simulink library "Loudness"  (R2022b)
settings: Solver=VariableStepAuto  StartTime=0.0  StopTime=10.0  RelTol=1e-3
InitFcn:
  | Loudness_init;
values from neighbouring files (symbols this model uses):
  COMP = struct('zipCoef', COMP_zipCoef,      'LoudBPFNum', COMPBASS_Num, 'LoudBPFDenom', COMPBASS_Denom,      'LoudLPFNum', COMPMID_Num, 'LoudLPFDenom', COMPMID_Denom,      'LoudBPFFreq',COMPBASS_Fc,'LoudBPFQ',COMPBASS_Q,      'LoudLPFFreq',COMPMID_Fc,'LoudLPFQ',COMPMID_Q)    [Loudness_init.m]
undefined symbols (not defined in the file or in its folder): dfilt, LOUD_BASS_0DB_SCALE, LOUD_BASS_D1, LOUD_BASS_D2, sys_defs
libraries: TuneVar x38, RTC x16, dspobslib x5
(part 2 of 2)

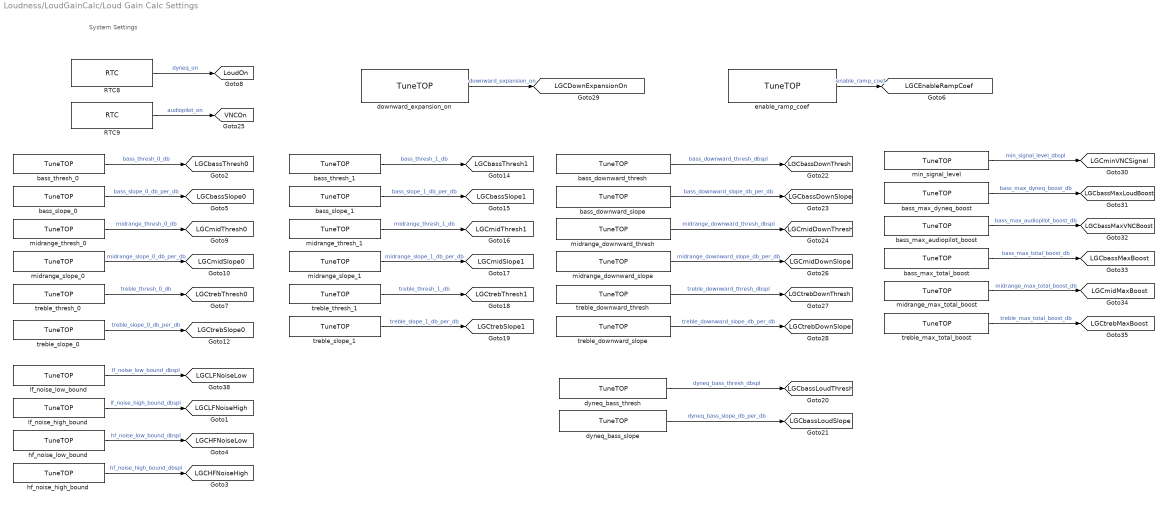
== system Loudness/LoudGainCalc/Loud Gain Calc Settings ==
  note: System Settings
  RTC8 : RTC/RTC  REQ_Priority=RTC_Mask.NormalPriority  RequestAtInit=off  EnableRequest=off  REQElemName1=dyneq_on  REQElemType1=single  REQElemWidth1=1  REQElemInitial1=[]  REQElemType2=single  REQElemWidth2=1  REQElemInitial2=[]  REQElemType3=uint32  REQElemWidth3=1  REQElemInitial3=[]  REQElemType4=uint32  REQElemWidth4=1  REQElemInitial4=[]  REQElemType5=uint32  REQElemWidth5=1  REQElemInitial5=[]  REQElemType6=uint32  REQElemWidth6=1  REQElemInitial6=[]  REQElemType7=uint32  REQElemWidth7=1  REQElemInitial7=[]  REQElemType8=uint32  REQElemWidth8=1  REQElemInitial8=[]  REQElemType9=uint32  REQElemWidth9=1  REQElemInitial9=[]  REQElemType10=uint32  REQElemWidth10=1  REQElemInitial10=[]  EnableResponse=off  EnableRSP_StatusIn=off  RSPElemType1=uint32  RSPElemWidth1=1  RSPElemType2=uint32  RSPElemWidth2=1  RSPElemType3=uint32  RSPElemWidth3=1  RSPElemType4=uint32  RSPElemWidth4=1  RSPElemType5=uint32  RSPElemWidth5=1  RSPElemType6=uint32  RSPElemWidth6=1  RSPElemType7=uint32  RSPElemWidth7=1  RSPElemType8=uint32  RSPElemWidth8=1  RSPElemType9=uint32  RSPElemWidth9=1  RSPElemType10=uint32  RSPElemWidth10=1  EnableNotification=off  EnableNTF_PrepTrig=off  NTFElemType1=uint32  NTFElemWidth1=1  NTFElemType2=uint32  NTFElemWidth2=1  NTFElemType3=uint32  NTFElemWidth3=1  NTFElemType4=uint32  NTFElemWidth4=1  NTFElemType5=uint32  NTFElemWidth5=1  NTFElemType6=uint32  NTFElemWidth6=1  NTFElemType7=uint32  NTFElemWidth7=1  NTFElemType8=uint32  NTFElemWidth8=1  NTFElemType9=uint32  NTFElemWidth9=1  NTFElemType10=uint32  NTFElemWidth10=1  MaskMessageName=setDyneqOn
  RTC9 : RTC/RTC  REQ_Priority=RTC_Mask.NormalPriority  RequestAtInit=off  EnableRequest=off  REQElemName1=audiopilot_on  REQElemType1=single  REQElemWidth1=1  REQElemInitial1=[]  REQElemType2=single  REQElemWidth2=1  REQElemInitial2=[]  REQElemType3=uint32  REQElemWidth3=1  REQElemInitial3=[]  REQElemType4=uint32  REQElemWidth4=1  REQElemInitial4=[]  REQElemType5=uint32  REQElemWidth5=1  REQElemInitial5=[]  REQElemType6=uint32  REQElemWidth6=1  REQElemInitial6=[]  REQElemType7=uint32  REQElemWidth7=1  REQElemInitial7=[]  REQElemType8=uint32  REQElemWidth8=1  REQElemInitial8=[]  REQElemType9=uint32  REQElemWidth9=1  REQElemInitial9=[]  REQElemType10=uint32  REQElemWidth10=1  REQElemInitial10=[]  EnableResponse=off  EnableRSP_StatusIn=off  RSPElemType1=uint32  RSPElemWidth1=1  RSPElemType2=uint32  RSPElemWidth2=1  RSPElemType3=uint32  RSPElemWidth3=1  RSPElemType4=uint32  RSPElemWidth4=1  RSPElemType5=uint32  RSPElemWidth5=1  RSPElemType6=uint32  RSPElemWidth6=1  RSPElemType7=uint32  RSPElemWidth7=1  RSPElemType8=uint32  RSPElemWidth8=1  RSPElemType9=uint32  RSPElemWidth9=1  RSPElemType10=uint32  RSPElemWidth10=1  EnableNotification=off  EnableNTF_PrepTrig=off  NTFElemType1=uint32  NTFElemWidth1=1  NTFElemType2=uint32  NTFElemWidth2=1  NTFElemType3=uint32  NTFElemWidth3=1  NTFElemType4=uint32  NTFElemWidth4=1  NTFElemType5=uint32  NTFElemWidth5=1  NTFElemType6=uint32  NTFElemWidth6=1  NTFElemType7=uint32  NTFElemWidth7=1  NTFElemType8=uint32  NTFElemWidth8=1  NTFElemType9=uint32  NTFElemWidth9=1  NTFElemType10=uint32  NTFElemWidth10=1  MaskMessageName=setAudioPilotOn
  bass_downward_slope : TuneVar/TuneTOP  TriggerInit=[-60 184 115 216]  TopName=bass_downward_slope_db_per_db  TuneName=bass_downward_slope_db_per_db  DataType=Inherit: Same as input  PackageName=mode  BankNumber=0  TunabilityNumber=1  MinValue=[]  MaxValue=[]  UseSameName=on  MaskValue=single([LGC.bassDownSlope])
  bass_downward_thresh : TuneVar/TuneTOP  TriggerInit=[-60 135 115 165]  TopName=bass_downward_thresh_dbspl  TuneName=bass_downward_thresh_dbspl  DataType=Inherit: Same as input  PackageName=mode  BankNumber=0  TunabilityNumber=1  MinValue=[]  MaxValue=[]  UseSameName=on  MaskValue=single([LGC.bassDownThresh])
  bass_max_audiopilot_boost : TuneVar/TuneTOP  TriggerInit=[445 230 605 260]  TopName=bass_max_audiopilot_boost_db  TuneName=bass_max_audiopilot_boost_db  DataType=Inherit: Same as input  PackageName=mode  BankNumber=0  TunabilityNumber=1  MinValue=[]  MaxValue=[]  UseSameName=on  MaskValue=single([LGC.bassMaxVNCBoost])
  bass_max_dyneq_boost : TuneVar/TuneTOP  TriggerInit=[445 179 605 211]  TopName=bass_max_dyneq_boost_db  TuneName=bass_max_dyneq_boost_db  DataType=Inherit: Same as input  PackageName=mode  BankNumber=0  TunabilityNumber=1  MinValue=[]  MaxValue=[]  UseSameName=on  MaskValue=single([LGC.bassMaxLoudBoost])
  bass_max_total_boost : TuneVar/TuneTOP  TriggerInit=[445 279 605 311]  TopName=bass_max_total_boost_db  TuneName=bass_max_total_boost_db  DataType=Inherit: Same as input  PackageName=mode  BankNumber=0  TunabilityNumber=1  MinValue=[]  MaxValue=[]  UseSameName=on  MaskValue=single([LGC.bassMaxBoost])
  bass_slope_0 : TuneVar/TuneTOP  TriggerInit=[-895 185 -755 215]  TopName=bass_slope_0_db_per_db  TuneName=bass_slope_0_db_per_db  DataType=Inherit: Same as input  PackageName=mode  BankNumber=0  TunabilityNumber=1  MinValue=[]  MaxValue=[]  UseSameName=on  MaskValue=single([LGC.bassSlope0])
  bass_slope_1 : TuneVar/TuneTOP  TriggerInit=[-470 185 -330 215]  TopName=bass_slope_1_db_per_db  TuneName=bass_slope_1_db_per_db  DataType=Inherit: Same as input  PackageName=mode  BankNumber=0  TunabilityNumber=1  MinValue=[]  MaxValue=[]  UseSameName=on  MaskValue=single([LGC.bassSlope1])
  bass_thresh_0 : TuneVar/TuneTOP  TriggerInit=[-895 135 -755 165]  TopName=bass_thresh_0_db  TuneName=bass_thresh_0_db  DataType=Inherit: Same as input  PackageName=mode  BankNumber=0  TunabilityNumber=1  MinValue=[]  MaxValue=[]  UseSameName=on  MaskValue=single([LGC.bassThresh0])
  bass_thresh_1 : TuneVar/TuneTOP  TriggerInit=[-470 135 -330 165]  TopName=bass_thresh_1_db  TuneName=bass_thresh_1_db  DataType=Inherit: Same as input  PackageName=mode  BankNumber=0  TunabilityNumber=1  MinValue=[]  MaxValue=[]  UseSameName=on  MaskValue=single([LGC.bassThresh1])
  downward_expansion_on : TuneVar/TuneTOP  TriggerInit=[-360 5 -195 55]  TopName=downward_expansion_on  TuneName=downward_expansion_on  DataType=Inherit: Same as input  PackageName=mode  BankNumber=0  TunabilityNumber=1  MinValue=[]  MaxValue=[]  UseSameName=on  MaskValue=single([LGC.downward_expansion_on])
  dyneq_bass_slope : TuneVar/TuneTOP  TriggerInit=[-55 529 110 561]  TopName=dyneq_bass_slope_db_per_db  TuneName=dyneq_bass_slope_db_per_db  DataType=Inherit: Same as input  PackageName=mode  BankNumber=0  TunabilityNumber=1  MinValue=[]  MaxValue=[]  UseSameName=on  MaskValue=single([LGC.bassLoudSlope])
  dyneq_bass_thresh : TuneVar/TuneTOP  TriggerInit=[-55 479 110 511]  TopName=dyneq_bass_thresh_dbspl  TuneName=dyneq_bass_thresh_dbspl  DataType=Inherit: Same as input  PackageName=mode  BankNumber=0  TunabilityNumber=1  MinValue=[]  MaxValue=[]  UseSameName=on  MaskValue=single([LGC.bassLoudThresh])
  enable_ramp_coef : TuneVar/TuneTOP  TriggerInit=[205 5 370 55]  TopName=enable_ramp_coef  TuneName=enable_ramp_coef  DataType=Inherit: Same as input  PackageName=mode  BankNumber=0  TunabilityNumber=1  MinValue=[]  MaxValue=[]  UseSameName=on  MaskValue=single(LGC.enableRampCoef)
  hf_noise_high_bound : TuneVar/TuneTOP  TriggerInit=[-895 610 -755 640]  TopName=hf_noise_high_bound_dbspl  TuneName=hf_noise_high_bound_dbspl  DataType=Inherit: Same as input  PackageName=mode  BankNumber=0  TunabilityNumber=1  MinValue=[]  MaxValue=[]  UseSameName=on  MaskValue=single([LGC.HFNoiseHigh])
  hf_noise_low_bound : TuneVar/TuneTOP  TriggerInit=[-895 560 -755 590]  TopName=hf_noise_low_bound_dbspl  TuneName=hf_noise_low_bound_dbspl  DataType=Inherit: Same as input  PackageName=mode  BankNumber=0  TunabilityNumber=1  MinValue=[]  MaxValue=[]  UseSameName=on  MaskValue=single([LGC.HFNoiseLow])
  lf_noise_high_bound : TuneVar/TuneTOP  TriggerInit=[-895 510 -755 540]  TopName=lf_noise_high_bound_dbspl  TuneName=lf_noise_high_bound_dbspl  DataType=Inherit: Same as input  PackageName=mode  BankNumber=0  TunabilityNumber=1  MinValue=[]  MaxValue=[]  UseSameName=on  MaskValue=single([LGC.LFNoiseHigh])
  lf_noise_low_bound : TuneVar/TuneTOP  TriggerInit=[-895 460 -755 490]  TopName=lf_noise_low_bound_dbspl  TuneName=lf_noise_low_bound_dbspl  DataType=Inherit: Same as input  PackageName=mode  BankNumber=0  TunabilityNumber=1  MinValue=[]  MaxValue=[]  UseSameName=on  MaskValue=single([LGC.LFNoiseLow])
  midrange_downward_slope : TuneVar/TuneTOP  TriggerInit=[-60 285 115 315]  TopName=midrange_downward_slope_db_per_db  TuneName=midrange_downward_slope_db_per_db  DataType=Inherit: Same as input  PackageName=mode  BankNumber=0  TunabilityNumber=1  MinValue=[]  MaxValue=[]  UseSameName=on  MaskValue=single([LGC.midDownSlope])
  midrange_downward_thresh : TuneVar/TuneTOP  TriggerInit=[-60 234 115 266]  TopName=midrange_downward_thresh_dbspl  TuneName=midrange_downward_thresh_dbspl  DataType=Inherit: Same as input  PackageName=mode  BankNumber=0  TunabilityNumber=1  MinValue=[]  MaxValue=[]  UseSameName=on  MaskValue=single([LGC.midDownThresh])
  midrange_max_total_boost : TuneVar/TuneTOP  TriggerInit=[445 331 605 359]  TopName=midrange_max_total_boost_db  TuneName=midrange_max_total_boost_db  DataType=Inherit: Same as input  PackageName=mode  BankNumber=0  TunabilityNumber=1  MinValue=[]  MaxValue=[]  UseSameName=on  MaskValue=single([LGC.midMaxBoost])
  midrange_slope_0 : TuneVar/TuneTOP  TriggerInit=[-895 285 -755 315]  TopName=midrange_slope_0_db_per_db  TuneName=midrange_slope_0_db_per_db  DataType=Inherit: Same as input  PackageName=mode  BankNumber=0  TunabilityNumber=1  MinValue=[]  MaxValue=[]  UseSameName=on  MaskValue=single([LGC.midSlope0])
  midrange_slope_1 : TuneVar/TuneTOP  TriggerInit=[-470 285 -330 315]  TopName=midrange_slope_1_db_per_db  TuneName=midrange_slope_1_db_per_db  DataType=Inherit: Same as input  PackageName=mode  BankNumber=0  TunabilityNumber=1  MinValue=[]  MaxValue=[]  UseSameName=on  MaskValue=single([LGC.midSlope1])
  midrange_thresh_0 : TuneVar/TuneTOP  TriggerInit=[-895 235 -755 265]  TopName=midrange_thresh_0_db  TuneName=midrange_thresh_0_db  DataType=Inherit: Same as input  PackageName=mode  BankNumber=0  TunabilityNumber=1  MinValue=[]  MaxValue=[]  UseSameName=on  MaskValue=single([LGC.midThresh0])
  midrange_thresh_1 : TuneVar/TuneTOP  TriggerInit=[-470 235 -330 265]  TopName=midrange_thresh_1_db  TuneName=midrange_thresh_1_db  DataType=Inherit: Same as input  PackageName=mode  BankNumber=0  TunabilityNumber=1  MinValue=[]  MaxValue=[]  UseSameName=on  MaskValue=single([LGC.midThresh1])
  min_signal_level : TuneVar/TuneTOP  TriggerInit=[445 131 605 159]  TopName=min_signal_level_dbspl  TuneName=min_signal_level_dbspl  DataType=Inherit: Same as input  PackageName=mode  BankNumber=0  TunabilityNumber=1  MinValue=[]  MaxValue=[]  UseSameName=on  MaskValue=single([LGC.minVNCSignal])
  treble_downward_slope : TuneVar/TuneTOP  TriggerInit=[-60 385 115 415]  TopName=treble_downward_slope_db_per_db  TuneName=treble_downward_slope_db_per_db  DataType=Inherit: Same as input  PackageName=mode  BankNumber=0  TunabilityNumber=1  MinValue=[]  MaxValue=[]  UseSameName=on  MaskValue=single([LGC.trebDownSlope])
  treble_downward_thresh : TuneVar/TuneTOP  TriggerInit=[-60 336 115 364]  TopName=treble_downward_thresh_dbspl  TuneName=treble_downward_thresh_dbspl  DataType=Inherit: Same as input  PackageName=mode  BankNumber=0  TunabilityNumber=1  MinValue=[]  MaxValue=[]  UseSameName=on  MaskValue=single([LGC.trebDownThresh])
  treble_max_total_boost : TuneVar/TuneTOP  TriggerInit=[445 380 605 410]  TopName=treble_max_total_boost_db  TuneName=treble_max_total_boost_db  DataType=Inherit: Same as input  PackageName=mode  BankNumber=0  TunabilityNumber=1  MinValue=[]  MaxValue=[]  UseSameName=on  MaskValue=single([LGC.trebMaxBoost])
  treble_slope_0 : TuneVar/TuneTOP  TriggerInit=[-895 390 -755 420]  TopName=treble_slope_0_db_per_db  TuneName=treble_slope_0_db_per_db  DataType=Inherit: Same as input  PackageName=mode  BankNumber=0  TunabilityNumber=1  MinValue=[]  MaxValue=[]  UseSameName=on  MaskValue=single([LGC.trebSlope0])
  treble_slope_1 : TuneVar/TuneTOP  TriggerInit=[-470 385 -330 415]  TopName=treble_slope_1_db_per_db  TuneName=treble_slope_1_db_per_db  DataType=Inherit: Same as input  PackageName=mode  BankNumber=0  TunabilityNumber=1  MinValue=[]  MaxValue=[]  UseSameName=on  MaskValue=single([LGC.trebSlope1])
  treble_thresh_0 : TuneVar/TuneTOP  TriggerInit=[-895 335 -755 365]  TopName=treble_thresh_0_db  TuneName=treble_thresh_0_db  DataType=Inherit: Same as input  PackageName=mode  BankNumber=0  TunabilityNumber=1  MinValue=[]  MaxValue=[]  UseSameName=on  MaskValue=single([LGC.trebThresh0])
  treble_thresh_1 : TuneVar/TuneTOP  TriggerInit=[-470 335 -330 365]  TopName=treble_thresh_1_db  TuneName=treble_thresh_1_db  DataType=Inherit: Same as input  PackageName=mode  BankNumber=0  TunabilityNumber=1  MinValue=[]  MaxValue=[]  UseSameName=on  MaskValue=single([LGC.trebThresh1])
  tag scope: LGCDownExpansionOn=global, LGCEnableRampCoef=global, LGCHFNoiseHigh=global, LGCHFNoiseLow=global, LGCLFNoiseHigh=global, LGCLFNoiseLow=global, LGCbassDownSlope=global, LGCbassDownThresh=global, LGCbassLoudSlope=global, LGCbassLoudThresh=global, LGCbassMaxBoost=global, LGCbassMaxLoudBoost=global, LGCbassMaxVNCBoost=global, LGCbassSlope0=global, LGCbassSlope1=global, LGCbassThresh0=global, LGCbassThresh1=global, LGCmidDownSlope=global, LGCmidDownThresh=global, LGCmidMaxBoost=global, LGCmidSlope0=global, LGCmidSlope1=global, LGCmidThresh0=global, LGCmidThresh1=global, LGCminVNCSignal=global, LGCtrebDownSlope=global, LGCtrebDownThresh=global, LGCtrebMaxBoost=global, LGCtrebSlope0=global, LGCtrebSlope1=global, LGCtrebThresh0=global, LGCtrebThresh1=global, LoudOn=global, VNCOn=global
  wires:
  lf_noise_low_bound/1 -> [LGCLFNoiseLow]  "lf_noise_low_bound_dbspl"
  lf_noise_high_bound/1 -> [LGCLFNoiseHigh]  "lf_noise_high_bound_dbspl"
  bass_thresh_0/1 -> [LGCbassThresh0]  "bass_thresh_0_db"
  bass_slope_0/1 -> [LGCbassSlope0]  "bass_slope_0_db_per_db"
  treble_thresh_0/1 -> [LGCtrebThresh0]  "treble_thresh_0_db"
  midrange_thresh_0/1 -> [LGCmidThresh0]  "midrange_thresh_0_db"
  midrange_slope_0/1 -> [LGCmidSlope0]  "midrange_slope_0_db_per_db"
  treble_slope_0/1 -> [LGCtrebSlope0]  "treble_slope_0_db_per_db"
  bass_thresh_1/1 -> [LGCbassThresh1]  "bass_thresh_1_db"
  bass_slope_1/1 -> [LGCbassSlope1]  "bass_slope_1_db_per_db"
  midrange_thresh_1/1 -> [LGCmidThresh1]  "midrange_thresh_1_db"
  midrange_slope_1/1 -> [LGCmidSlope1]  "midrange_slope_1_db_per_db"
  treble_slope_1/1 -> [LGCtrebSlope1]  "treble_slope_1_db_per_db"
  dyneq_bass_thresh/1 -> [LGCbassLoudThresh]  "dyneq_bass_thresh_dbspl"
  dyneq_bass_slope/1 -> [LGCbassLoudSlope]  "dyneq_bass_slope_db_per_db"
  bass_downward_thresh/1 -> [LGCbassDownThresh]  "bass_downward_thresh_dbspl"
  bass_downward_slope/1 -> [LGCbassDownSlope]  "bass_downward_slope_db_per_db"
  midrange_downward_thresh/1 -> [LGCmidDownThresh]  "midrange_downward_thresh_dbspl"
  midrange_downward_slope/1 -> [LGCmidDownSlope]  "midrange_downward_slope_db_per_db"
  treble_downward_thresh/1 -> [LGCtrebDownThresh]  "treble_downward_thresh_dbspl"
  treble_downward_slope/1 -> [LGCtrebDownSlope]  "treble_downward_slope_db_per_db"
  min_signal_level/1 -> [LGCminVNCSignal]  "min_signal_level_dbspl"
  bass_max_dyneq_boost/1 -> [LGCbassMaxLoudBoost]  "bass_max_dyneq_boost_db"
  bass_max_audiopilot_boost/1 -> [LGCbassMaxVNCBoost]  "bass_max_audiopilot_boost_db"
  bass_max_total_boost/1 -> [LGCbassMaxBoost]  "bass_max_total_boost_db"
  midrange_max_total_boost/1 -> [LGCmidMaxBoost]  "midrange_max_total_boost_db"
  treble_max_total_boost/1 -> [LGCtrebMaxBoost]  "treble_max_total_boost_db"
  downward_expansion_on/1 -> [LGCDownExpansionOn]  "downward_expansion_on"
  treble_thresh_1/1 -> [LGCtrebThresh1]  "treble_thresh_1_db"
  hf_noise_low_bound/1 -> [LGCHFNoiseLow]  "hf_noise_low_bound_dbspl"
  hf_noise_high_bound/1 -> [LGCHFNoiseHigh]  "hf_noise_high_bound_dbspl"
  RTC8/1 -> [LoudOn]  "dyneq_on"
  RTC9/1 -> [VNCOn]  "audiopilot_on"
  enable_ramp_coef/1 -> [LGCEnableRampCoef]  "enable_ramp_coef"

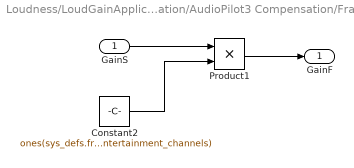
== system Loudness/LoudGainApplication/AudioPilot3 Compensation/Framify ==
  GainS : Inport
  Constant2 : Constant  Value=ones(sys_defs.frameSize, sys_defs.number_of_input_entertainment_channels)  VectorParams1D=off  OutDataTypeStr=single
  Product1 : Product  RndMeth=Zero
  GainF : Outport  VectorParamsAs1DForOutWhenUnconnected=off
  wires:
  Product1/1 -> GainF/1
  Constant2/1 -> Product1/2
  GainS/1 -> Product1/1

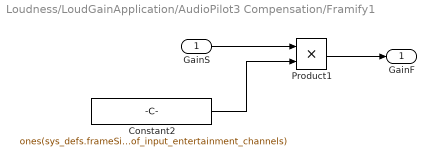
== system Loudness/LoudGainApplication/AudioPilot3 Compensation/Framify1 ==
  GainS : Inport  OutDataTypeStr=single
  Constant2 : Constant  Value=ones(sys_defs.frameSize, sys_defs.number_of_input_entertainment_channels)  VectorParams1D=off  OutDataTypeStr=single
  Product1 : Product  RndMeth=Zero
  GainF : Outport  VectorParamsAs1DForOutWhenUnconnected=off
  wires:
  GainS/1 -> Product1/1
  Constant2/1 -> Product1/2
  Product1/1 -> GainF/1

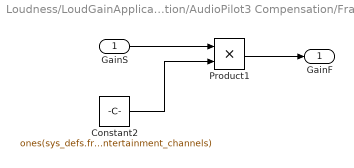
== system Loudness/LoudGainApplication/AudioPilot3 Compensation/Framify2 ==
  GainS : Inport
  Constant2 : Constant  Value=ones(sys_defs.frameSize, sys_defs.number_of_input_entertainment_channels)  VectorParams1D=off  OutDataTypeStr=single
  Product1 : Product  RndMeth=Zero
  GainF : Outport  VectorParamsAs1DForOutWhenUnconnected=off
  wires:
  Product1/1 -> GainF/1
  Constant2/1 -> Product1/2
  GainS/1 -> Product1/1

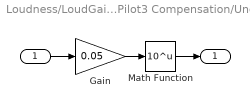
== system Loudness/LoudGainApplication/AudioPilot3 Compensation/UndB ==
  " " : Inport
  Gain : Gain  Gain=0.05  SaturateOnIntegerOverflow=on  OutDataTypeStr=Inherit: Same as input  ParamDataTypeStr=Inherit: Same as input
  Math Function : Math  Operator=10^u  SignedPower=on
  "  " : Outport  VectorParamsAs1DForOutWhenUnconnected=off
  wires:
  Gain/1 -> Math Function/1
  Math Function/1 -> "  "/1
  " "/1 -> Gain/1

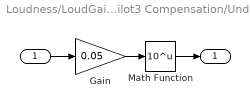
== system Loudness/LoudGainApplication/AudioPilot3 Compensation/UndB1 ==
  " " : Inport
  Gain : Gain  Gain=0.05  SaturateOnIntegerOverflow=on  OutDataTypeStr=Inherit: Same as input  ParamDataTypeStr=Inherit: Same as input
  Math Function : Math  Operator=10^u  SignedPower=on
  "  " : Outport  VectorParamsAs1DForOutWhenUnconnected=off
  wires:
  " "/1 -> Gain/1
  Math Function/1 -> "  "/1
  Gain/1 -> Math Function/1

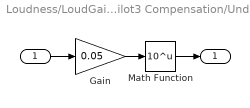
== system Loudness/LoudGainApplication/AudioPilot3 Compensation/UndB2 ==
  " " : Inport
  Gain : Gain  Gain=0.05  SaturateOnIntegerOverflow=on  OutDataTypeStr=Inherit: Same as input  ParamDataTypeStr=Inherit: Same as input
  Math Function : Math  Operator=10^u  SignedPower=on
  "  " : Outport  VectorParamsAs1DForOutWhenUnconnected=off
  wires:
  " "/1 -> Gain/1
  Math Function/1 -> "  "/1
  Gain/1 -> Math Function/1

== matlab function Loudness/LoudGainCalc/Boost Map Adjustments ==
  data: Bthresh output; Bslope output; noise input; LFNoiseLow input; LFNoiseHigh input; HFNoiseLow input; HFNoiseHigh input; ratio input; ratioLow input; ratioHigh input; BT0 input; BS0 input; MT0 input; MS0 input; TT0 input; TS0 input; BT1 input; BS1 input; MT1 input; MS1 input; TT1 input; Mthresh output; Mslope output; TS1 input; Tthresh output; Tslope output; HFNoise input
function [Bthresh, Bslope, Mthresh, Mslope, Tthresh ,Tslope] = ...
	fcn(noise, ...
	LFNoiseLow, LFNoiseHigh, ...
	HFNoiseLow, HFNoiseHigh, ...
    ratio, ratioLow, ratioHigh, ...
	BT0, BS0, MT0, MS0, TT0, TS0, ...
	BT1, BS1, MT1, MS1, TT1, TS1,HFNoise)
% This block supports an embeddable subset of the MATLAB language.
% See the help menu for details. 

% Initializing the parameters
% Concatenate ratioHigh & ratioLow to form ratio0
ratio0 = [ratioHigh ratioLow];
% Concatenate BT0 & BT1 to form Bthresh0
Bthresh0 = [BT0 BT1];
% Concatenate MT0 & MT1 to form Mthresh0
Mthresh0 = [MT0 MT1];
% Concatenate TT0 & TT1 to form Tthresh0
Tthresh0 = [TT0 TT1];
% Concatenate BS0 & BS1 to form Bslope0
Bslope0 = [BS0 BS1];
% Concatenate MS0 & MS1 to form Mslope0
Mslope0 = [MS0 MS1];
% Concatenate TS0 & TS1 to form Tslope0
Tslope0 = [TS0 TS1];
% Assign Value for alpha based on HFNoise, HFNoiseLow & HFNoiseHigh values
if HFNoise < HFNoiseLow
    alpha = single(0);
elseif HFNoise > HFNoiseHigh
    alpha = single(1);
else
    alpha = single((HFNoise-HFNoiseLow)/(HFNoiseHigh-HFNoiseLow));
end
% Assign Value for beta based on noise, LFNoiseLow & LFNoiseHigh values
if noise < LFNoiseLow
    beta = single(0);
elseif noise > LFNoiseHigh
    beta = single(1);
else
    beta  = single((noise-LFNoiseLow)/(LFNoiseHigh-LFNoiseLow));
end

alpha = alpha * beta;

% Assign values for Bslope,Mslope,Tslope,Bthresh,Mthresh & Tthresh
% based on the values of ratio, ratioHigh and ratioLow
if ratio >= ratioHigh
    Bslope = (interp1(ratio0, Bslope0, ratioHigh, 'linear'))*alpha + (1-alpha)*Bslope0(1);
    Mslope = (interp1(ratio0, Mslope0, ratioHigh, 'linear'))*alpha + (1-alpha)*Mslope0(1);
    Tslope = (interp1(ratio0, Tslope0, ratioHigh, 'linear'))*alpha + (1-alpha)*Tslope0(1);
    Bthresh = (interp1(ratio0, Bthresh0, ratioHigh, 'linear'))*alpha + (1-alpha)*Bthresh0(1);
    Mthresh = (interp1(ratio0, Mthresh0, ratioHigh, 'linear'))*alpha + (1-alpha)*Mthresh0(1);
    Tthresh = (interp1(ratio0, Tthresh0, ratioHigh, 'linear'))*alpha + (1-alpha)*Tthresh0(1);
elseif (ratio > ratioLow) && (ratio < ratioHigh)
    Bslope = (interp1(ratio0, Bslope0, ratio, 'linear'))*alpha + (1-alpha)*Bslope0(1);
    Mslope = (interp1(ratio0, Mslope0, ratio, 'linear'))*alpha + (1-alpha)*Mslope0(1);
    Tslope = (interp1(ratio0, Tslope0, ratio, 'linear'))*alpha + (1-alpha)*Tslope0(1);
    Bthresh = (interp1(ratio0, Bthresh0, ratio, 'linear'))*alpha + (1-alpha)*Bthresh0(1);
    Mthresh = (interp1(ratio0, Mthresh0, ratio, 'linear'))*alpha + (1-alpha)*Mthresh0(1);
    Tthresh = (interp1(ratio0, Tthresh0, ratio, 'linear'))*alpha + (1-alpha)*Tthresh0(1);
else
    Bslope = (interp1(ratio0, Bslope0, ratioLow, 'linear'))*alpha + (1-alpha)*Bslope0(1);
    Mslope = (interp1(ratio0, Mslope0, ratioLow, 'linear'))*alpha + (1-alpha)*Mslope0(1);
    Tslope = (interp1(ratio0, Tslope0, ratioLow, 'linear'))*alpha + (1-alpha)*Tslope0(1);    
    Bthresh = (interp1(ratio0, Bthresh0, ratioLow, 'linear'))*alpha + (1-alpha)*Bthresh0(1);
    Mthresh = (interp1(ratio0, Mthresh0, ratioLow, 'linear'))*alpha + (1-alpha)*Mthresh0(1);
    Tthresh = (interp1(ratio0, Tthresh0, ratioLow, 'linear'))*alpha + (1-alpha)*Tthresh0(1); 
end

== matlab function Loudness/LoudGainCalc/MATLAB Function ==
  data: bassBoost input; boostAverage output; midBoost input; trebleBoost input; maxBassBoost input; maxMidBoost input; maxTrebleBoost input
  events: trigger input FUNCTION_CALL_EVENT
function boostAverage = getAverageAudioPilotBoostLevel(bassBoost, midBoost, trebleBoost, maxBassBoost, maxMidBoost, maxTrebleBoost)
% This function calculates the average boost value for a given set of bass,
% mid, and treble boost values. A boost value is included in the average if
% the corresponding maximum boost value is greater than a threshold.

cTHRESHOLD = single(1e-12);
cONE = single(1);
% Initializing the parameters
count = single(0);
divBass = single(0);
divMid = single(0);
divTreble = single(0);
% Check if maxBassBoost is greater than cTHRESHOLD
if (maxBassBoost > cTHRESHOLD) 
    divBass = bassBoost/maxBassBoost;
    count = count + 1;
end
% Check if maxMidBoost is greater than cTHRESHOLD
if (maxMidBoost > cTHRESHOLD) 
    divMid = midBoost/maxMidBoost;
    count = count + 1;
end
% Check if maxTrebleBoost is greater than cTHRESHOLD
if (maxTrebleBoost > cTHRESHOLD) 
    divTreble = trebleBoost/maxTrebleBoost;
    count = count + 1;
end

boostAverage = (divBass + divMid + divTreble);
% Check if count is greater than cONE
if (count > cONE)    
    boostAverage = boostAverage/count;
end

== matlab function Loudness/LoudGainCalc/NoiseOverRide ==
  data: LFNoiseIn input; LFNoiseOverRideFlag input; LFNoiseOverRide input; LFNoise output; WBNoiseIn input; WBNoiseOverRideFlag input; WBNoiseOverRide input; WBNoise output; HFNoiseIn input; HFNoiseOverRideFlag input; HFNoiseOverRide input; RatioIn input; RatioOverRideFlag input; RatioOverRide input; HFNoise output; Ratio output
function [LFNoise, WBNoise, HFNoise, Ratio] = ...
    OverRide(LFNoiseIn, LFNoiseOverRideFlag, LFNoiseOverRide, ...
            WBNoiseIn, WBNoiseOverRideFlag, WBNoiseOverRide, ...
            HFNoiseIn, HFNoiseOverRideFlag, HFNoiseOverRide,  ...
            RatioIn, RatioOverRideFlag, RatioOverRide )
% Initializing the parameters LFNoise, WBNoise, HFNoise & Ratio
LFNoise = LFNoiseIn;
WBNoise = WBNoiseIn;
HFNoise = HFNoiseIn;
Ratio = RatioIn;
% Check if LFNoiseOverRideFlag is enabled, if yes then reinitialize the
% value of LFNoise
if (LFNoiseOverRideFlag)
    LFNoise = LFNoiseOverRide;
end
% Check if WBNoiseOverRideFlag is enabled, if yes then reinitialize the
% value of WBNoise
if (WBNoiseOverRideFlag)
    WBNoise = WBNoiseOverRide;
end
% Check if HFNoiseOverRideFlag is enabled, if yes then reinitialize the
% value of HFNoise
if (HFNoiseOverRideFlag)
    HFNoise = HFNoiseOverRide;
end
% Check if RatioOverRideFlag is enabled, if yes then reinitialize the
% value of Ratio
if (RatioOverRideFlag)
    Ratio = RatioOverRide;
end

== matlab function Loudness/LoudGainCalc/ramperFcn ==
  data: dyneq_boost_gain output; vnc_boost_gain output; rampCoef input; loud_on input; VNC_on input
function [ dyneq_boost_gain, vnc_boost_gain] = fcn(rampCoef, loud_on, VNC_on)

persistent  dyneq_boost_gain_prev; 
persistent  vnc_boost_gain_prev;
% Assign dyneq_boost_gain_prev to zero if it is empty
if isempty(dyneq_boost_gain_prev) 
   dyneq_boost_gain_prev = single(0);
end
% Assign vnc_boost_gain_prev to zero if it is empty
if isempty(vnc_boost_gain_prev) 
   vnc_boost_gain_prev = single(0);
end
% Compute the values of dyneq_boost_gain 
dyneq_boost_gain = ((1-rampCoef) * loud_on) ...
                     + (rampCoef * dyneq_boost_gain_prev);
% Compute the values of  vnc_boost_gain
vnc_boost_gain = ((1-rampCoef) * VNC_on) ...
                     + (rampCoef * vnc_boost_gain_prev);
% update the dyneq_boost_gain_prev & vnc_boost_gain_prev variables                
dyneq_boost_gain_prev = dyneq_boost_gain;
vnc_boost_gain_prev = vnc_boost_gain;

== matlab function Loudness/LoudGainCalc/Gain Calculations ==
  data: bassBoost output; VNCSignal input; midBoost output; LoudSignal input; LFNoise input; WBNoise input; loud_on input; VNC_on input; bassVNCThresh input; bassVNCSlope input; midVNCThresh input; midVNCSlope input; trebleVNCThresh input; trebleVNCSlope input; minVNCSignal input =minVNCSignal; bassLoudThresh input =bassLoudThresh; bassLoudSlope input =bassLoudSlope; bassDownThresh input =bassDownThresh; bassDownSlope input =bassDownSlope; bassMaxLoudBoost input =bassMaxLoudBoost; bassMaxVNCBoost input =bassMaxVNCBoost; bassMaxBoost input =bassMaxBoost; midDownThresh input =midDownThresh; midDownSlope input =midDownSlope; midMaxBoost input =midMaxBoost; trebleDownThresh input; trebleDownSlope input; trebleMaxBoost input; trebleBoost output; downward_expansion_on input; LoudSignalOverRideFlag input; LoudSignalOverRide input; VNCSignalOverRideFlag input; VNCSignalOverRide input; VNCTrebleBoostOverRideFlag input; VNCTrebleBoostOverRide input; VNCMidBoostOverRideFlag input; VNCMidBoostOverRide input; VNCBassBoostOverRideFlag input; VNCBassBoostOverRide input; DynEQBoostOverRideFlag input; DynEQBoostOverRide input; dyneq_boost output; vnc_bass_boost output
function [bassBoost, midBoost, trebleBoost, dyneq_boost, vnc_bass_boost] ...
    = loudgaincalc(VNCSignal, LoudSignal, ...
    LFNoise, WBNoise, loud_on, VNC_on, ...
    bassVNCThresh, bassVNCSlope, midVNCThresh, midVNCSlope, ...
    trebleVNCThresh, trebleVNCSlope, minVNCSignal, ...
    bassLoudThresh, bassLoudSlope, bassDownThresh, bassDownSlope, ...
    bassMaxLoudBoost, bassMaxVNCBoost, bassMaxBoost, ...
    midDownThresh, midDownSlope, midMaxBoost, ...
    trebleDownThresh, trebleDownSlope, trebleMaxBoost,...
    downward_expansion_on, ...
    LoudSignalOverRideFlag, LoudSignalOverRide, ...
    VNCSignalOverRideFlag, VNCSignalOverRide, ...
    VNCTrebleBoostOverRideFlag, VNCTrebleBoostOverRide, ...
    VNCMidBoostOverRideFlag, VNCMidBoostOverRide, ...
    VNCBassBoostOverRideFlag, VNCBassBoostOverRide, ...
    DynEQBoostOverRideFlag, DynEQBoostOverRide)
% Check if LoudSignalOverRideFlag is enabled
if (LoudSignalOverRideFlag)
    LoudSignal = LoudSignalOverRide;
end
% Check if VNCSignalOverRideFlag is enabled
if (VNCSignalOverRideFlag)
    VNCSignal = VNCSignalOverRide;
else
    VNCSignal = max(VNCSignal, minVNCSignal);
end
% Check if VNCTrebleBoostOverRideFlag is enabled
if (VNCTrebleBoostOverRideFlag)
    trebleBoost = VNCTrebleBoostOverRide;
else
    % if not enabled then call vnc_boost function to compute the value
    % for trebleBoost
    trebleBoost = vnc_boost(VNCSignal, WBNoise, ...
        trebleVNCThresh, trebleVNCSlope, ...
        trebleDownThresh, trebleDownSlope, ...
        trebleMaxBoost, downward_expansion_on)*VNC_on;
end
% Check if VNCMidBoostOverRideFlag is enabled
if (VNCMidBoostOverRideFlag)
    midBoost = VNCMidBoostOverRide;
else
    % if not enabled then call vnc_boost function to compute the value
    % for midBoost
    midBoost = vnc_boost(VNCSignal, WBNoise, ...
        midVNCThresh, midVNCSlope, ...
        midDownThresh, midDownSlope, ...
        midMaxBoost, downward_expansion_on)*VNC_on;
end
% Check if VNCMidBoostOverRideFlag is enabled
if (VNCBassBoostOverRideFlag)
    vnc_bass_boost = VNCBassBoostOverRide;
else
    % if not enabled then call vnc_boost function to compute the value
    % for vnc_bass_boost
    vnc_bass_boost = vnc_boost(VNCSignal, LFNoise, ...
        bassVNCThresh, bassVNCSlope, ...
        bassDownThresh, bassDownSlope, ...
        bassMaxVNCBoost, downward_expansion_on)*VNC_on;
end
% Check if VNCMidBoostOverRideFlag is enabled
if (DynEQBoostOverRideFlag)
    dyneq_boost = DynEQBoostOverRide;
else
    % if not enabled then call loudness_boost function to compute the value
    % for dyneq_boost
    dyneq_boost = loudness_boost(LoudSignal+trebleBoost, ...
        bassLoudThresh, bassLoudSlope, ...
        bassMaxLoudBoost)*loud_on;
end
bassBoost = vnc_bass_boost + dyneq_boost ;
% Assign bassBoost to min among bassBoost& bassMaxBoost
bassBoost = min(bassBoost, bassMaxBoost);
% To find the boost value through loudness_boost function
function boost = loudness_boost(signal, threshold, slope, maximum)
boost = max((threshold- signal) * slope,0);
% Assign boost to min among boost & maximum
boost = min(boost,maximum);
return
% To find the boost value through vnc_boost function
function boost = vnc_boost(signal, noise, threshold, slope, down_thresh, down_slope, maximum, downward_expansion_on) %#ok<INUSD>
boost = (threshold+noise-signal)*slope;
% Check if down_slope is greater than zero
if (down_slope>0)
    boost = min(boost,(signal-down_thresh)*down_slope*downward_expansion_on);
end
% Assign boost to min among boost & zero
boost = max(boost,0);
% Now boost is min of boost and maximum
boost = min(boost,maximum);
return
